simulink model "Sfunction_stepback"  (R2021b)
settings: Solver=VariableStepAuto  StartTime=0.0  StopTime=40  RelTol=1e-3
libraries: simulink x1
settings Model: Creator=旧友  LastModifiedBy=旧友

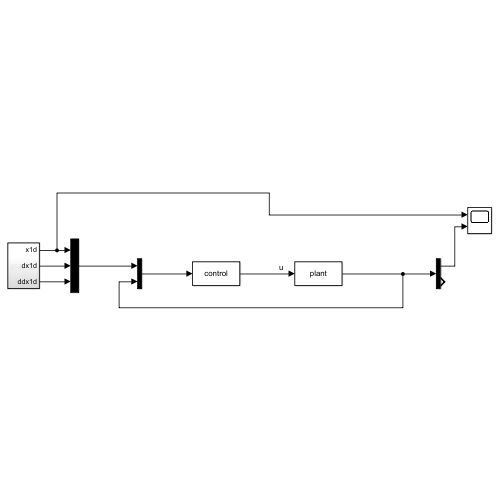
[thumbnail: Simulink's stored preview of the top-level diagram]
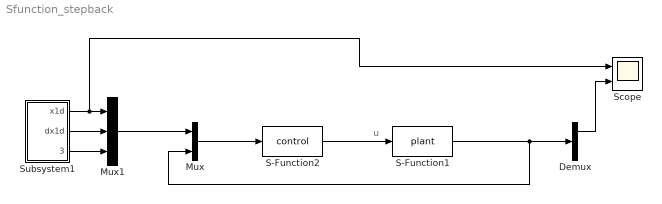
== system Sfunction_stepback ==
  note: u
  Demux : Demux  Outputs=2
  Mux : Mux  Inputs=2
  Mux1 : Mux  Inputs=3
  S-Function1 : S-Function  FunctionName=plant  Parameters=pa  SFunctionDeploymentMode=off  EnableBusSupport=off
  S-Function2 : S-Function  FunctionName=control  Parameters=pa  SFunctionDeploymentMode=off  EnableBusSupport=off
  Scope : Scope  NumInputPorts=2
  Subsystem1 : Subsystem
  wires:
  S-Function2/1 -> S-Function1/1
  S-Function1/1 -> Mux/2, Demux/1
  Demux/1 -> Scope/2
  Mux/1 -> S-Function2/1
  Subsystem1/1(x1d) -> Scope/1, Mux1/1
  Subsystem1/2(dx1d) -> Mux1/2
  Subsystem1/3(ddx1d) -> Mux1/3
  Mux1/1 -> Mux/1

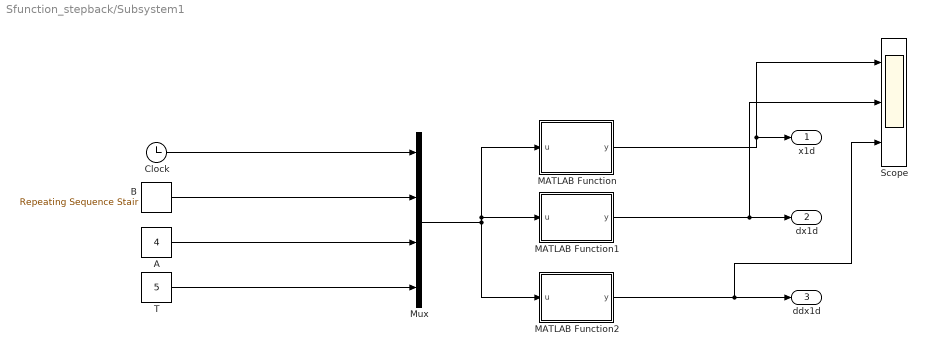
== system Sfunction_stepback/Subsystem1 ==
  A : Constant  Value=4
  B : simulink/Sources/Repeating Sequence Stair  OutValues=0  tsamp=20  OutMin=[]  OutMax=[]  OutDataTypeStr=double  OutputDataTypeScalingMode=double  OutDataType=fixdt(0,8)  ConRadixGroup=Best Precision: Vector-wise  OutScaling=2^-12
  Clock : Clock
      settings: Decimation=50
  MATLAB Function : MATLAB Function  TreatAsAtomicUnit=on
  MATLAB Function1 : MATLAB Function  TreatAsAtomicUnit=on
  MATLAB Function2 : MATLAB Function  TreatAsAtomicUnit=on
  Mux : Mux
  Scope : Scope  NumInputPorts=3
  T : Constant  Value=5
  x1d : Outport
  dx1d : Outport  Port=2
  ddx1d : Outport  Port=3
  wires:
  Clock/1 -> Mux/1
  B/1 -> Mux/2
  Mux/1 -> MATLAB Function/1(u), MATLAB Function1/1(u), MATLAB Function2/1(u)
  MATLAB Function/1(y) -> Scope/1, x1d/1
  MATLAB Function1/1(y) -> Scope/2, dx1d/1
  T/1 -> Mux/4
  MATLAB Function2/1(y) -> Scope/3, ddx1d/1
  A/1 -> Mux/3

== matlab function Sfunction_stepback/Subsystem1/MATLAB Function ==
  data: u input; y output
function y = fcn(u)
y = u(2)+u(3)*sin(2*pi/u(4)*u(1))

== matlab function Sfunction_stepback/Subsystem1/MATLAB Function1 ==
  data: u input; y output
function y = fcn(u)
y = 2*pi/u(4)*u(3)*cos(2*pi/u(4)*u(1));

== matlab function Sfunction_stepback/Subsystem1/MATLAB Function2 ==
  data: u input; y output
function y = fcn(u)
y = -4*pi*pi/u(4)/u(4)*u(3)*sin(2*pi/u(4)*u(1));
